simulink model "EKF"  (R2023b)
settings: Solver=FixedStepAuto  StartTime=12982  StopTime=20138  FixedStep=1  RelTol=1e-3
undefined symbols (not defined in the file or in its folder): Bat_Capacity, OCV_LUT, SOC_LUT
settings Model: Creator=Administrator  LastModifiedBy=Administrator

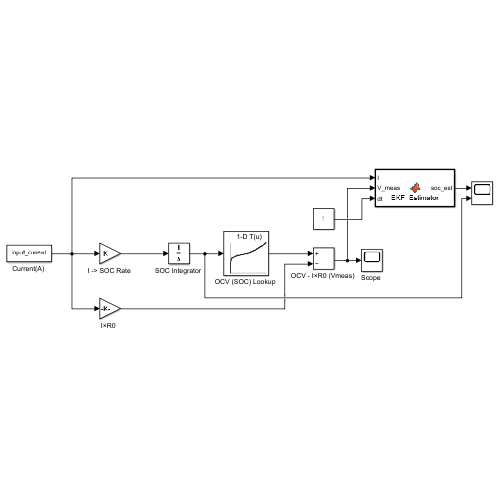
[thumbnail: Simulink's stored preview of the top-level diagram]
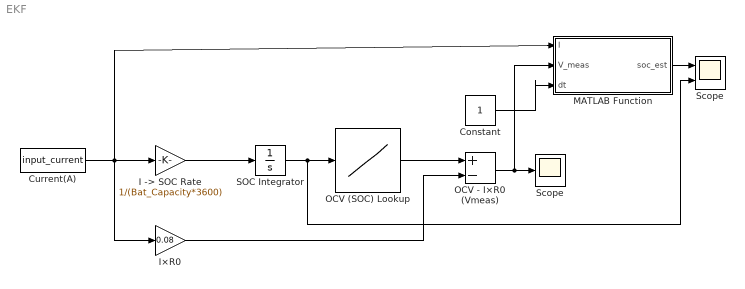
== system EKF ==
  Constant : Constant
  "Current(A) " : FromWorkspace  VariableName=input_current  OutDataTypeStr=double  SampleTime=1
  "I -> SOC Rate " : Gain  Gain=1/(Bat_Capacity*3600)
  "I×R0  " : Gain  Gain=0.08
  MATLAB Function : MATLAB Function  TreatAsAtomicUnit=on
  "OCV (SOC) Lookup " : Lookup_n-D  NumberOfTableDimensions=1  BreakpointsForDimension1=SOC_LUT  Table=OCV_LUT  InternalRulePriority=Speed  RndMeth=Simplest
  "OCV - I×R0 (Vmeas) " : Sum  Inputs=+-
  "SOC Integrator " : Integrator  InitialCondition=1
  Scope : Scope  NumInputPorts=2
  "Scope " : Scope
  wires:
  "Current(A) "/1 -> MATLAB Function/1(I), "I -> SOC Rate "/1, "I×R0  "/1
  "I -> SOC Rate "/1 -> "SOC Integrator "/1
  "SOC Integrator "/1 -> Scope/2, "OCV (SOC) Lookup "/1
  "OCV (SOC) Lookup "/1 -> "OCV - I×R0 (Vmeas) "/1
  "I×R0  "/1 -> "OCV - I×R0 (Vmeas) "/2
  "OCV - I×R0 (Vmeas) "/1 -> MATLAB Function/2(V_meas), "Scope "/1
  Constant/1 -> MATLAB Function/3(dt)
  MATLAB Function/1(soc_est) -> Scope/1

== matlab function EKF/MATLAB Function ==
  settings: updateMethod=DISCRETE
  data: I input; soc_est output; V_meas input; dt input
function soc_est = EKF_Estimator(I, V_meas, dt)
    % EKF SOC 估算器
    % 输入:
    %   I: 电流 (A), 放电为负 (注意你的数据定义，如果反了要加负号)
    %   V_meas: 测量电压 (V)
    %   dt: 采样时间 (s)
    % 输出:
    %   soc_est: 估算的 SOC

    % --- 1. 参数定义 (必须与对象模型一致，或者是辨识出的参数) ---
    % 为了演示简单，我们硬编码刚才的参数。
    % 实际项目中这些应该作为外部参数输入。
    R0 = 0.08;      % 欧姆内阻
    Qn = 2.0;       % 额定容量 (Ah)，这里填你刚才算出的 Bat_Capacity 约数
    Capacity = Qn * 3600; % 转为安时秒

    % 过程噪声 (Q) 和 观测噪声 (R) - 调参的关键！
    Q_cov = 1e-5;   % 认为安时积分很准，但有微小误差
    R_cov = 0.1;    % 认为电压测量有 0.1V 左右的波动

    % --- 2. 状态存储 (Persistent 变量在函数调用间保持值) ---
    persistent x_hat P
    if isempty(x_hat)
        x_hat = 1; % <--- 【关键】故意设一个错误的初始值(比如80%)，看它能不能自动收敛到100%
        P = 0.1;     % 初始协方差
    end

    % --- 3. 状态预测 (Time Update) ---
    % 安时积分预测 SOC
    % SOC_k = SOC_{k-1} + (I * dt / Capacity)
    % 注意：如果你的电流放电是负数，这里应该是加号。
    x_pred = x_hat + (I * dt / Capacity); 
    
    % 预测协方差
    P_pred = P + Q_cov;

    % --- 4. 测量更新 (Measurement Update) ---
    % 计算雅可比矩阵 H = d(OCV)/d(SOC)
    % 这里我们需要查表得到当前的 OCV 以及 OCV 对 SOC 的斜率
    % 简单做法：利用查表函数 (coder.extrinsic 声明外部函数，或者简化处理)
    
    % 为了能在 MATLAB Function 里查表，我们用简化的 5阶多项式拟合 OCV
    % (实际工程中建议把 Look-up Table 放在外部，传入 OCV 值)
    % 这里我们用一个简易线性假设演示原理：在 3.0-4.2V 区间，OCV 近似线性
    % OCV_pred ≈ 3.0 + 1.2 * x_pred
    % 实际上你应该用 polyfit 提前拟合好系数: p = polyfit(SOC_Vector, OCV_Vector, 6);
    % OCV_pred = polyval(p, x_pred);
    
    % 为了不让你报错，我们先假设一个简单的 OCV 关系用于调试代码逻辑：
    OCV_pred = 3.2 + (4.2 - 3.2) * x_pred; 
    dOCV_dSOC = (4.2 - 3.2); % 斜率 H

    % 预测端电压
    V_pred = OCV_pred + I * R0; % 注意符号：放电I为负，V端 = OCV + I*R (如果不确定，看电压是不是比OCV低)

    % 计算卡尔曼增益
    H = dOCV_dSOC;
    K = P_pred * H' / (H * P_pred * H' + R_cov);

    % 更新状态 (校正 SOC)
    innovation = V_meas - V_pred; % 观测误差
    x_hat = x_pred + K * innovation;
    
    % 更新协方差
    P = (1 - K * H) * P_pred;

    % --- 5. 输出 ---
    soc_est = x_hat;
end
